simulink model "Russia"  (R2024a)
settings: Solver=VariableStepAuto  StartTime=0.0  StopTime=10.0  RelTol=1e-3
libraries: fuzblock x1
settings Model: Creator=Тимур  LastModifiedBy=Тимур

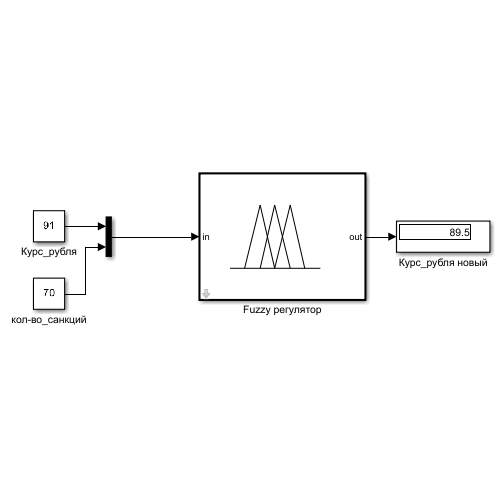
[thumbnail: Simulink's stored preview of the top-level diagram]
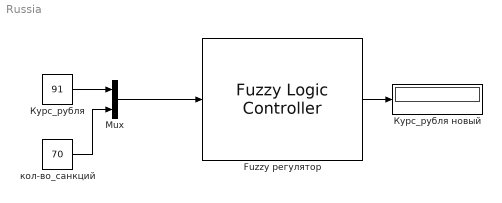
== system Russia ==
  Fuzzy регулятор : fuzblock/Fuzzy Logic  Controller  FIS='C:/Users/Тимур/Документы/MATLAB/Laba9_10/Zadanie5.fis'  OutputSampleNumber=101  DataType=double  FuzzifiedInputs=off  RuleFiringStrengths=off  RuleOutputs=off  AggregatedOutputs=off  SimulateUsing=Interpreted execution  OutOfRangeInputValueMessage=warning  NoRuleFiredMessage=warning  EmptyOutputFuzzySetMessage=warning
  Mux : Mux  Inputs=2
  Курс_рубля : Constant  Value=91
  Курс_рубля новый : Display
  кол-во_санкций : Constant  Value=70
  wires:
  Курс_рубля/1 -> Mux/1
  кол-во_санкций/1 -> Mux/2
  Mux/1 -> Fuzzy регулятор/1
  Fuzzy регулятор/1 -> Курс_рубля новый/1
